simulink subsystem "Control_Motores"  (R2023b)
settings: Solver=VariableStepAuto  StartTime=0.0  StopTime=10.0  RelTol=1e-3
settings Model: Creator=Felix  LastModifiedBy=Felix

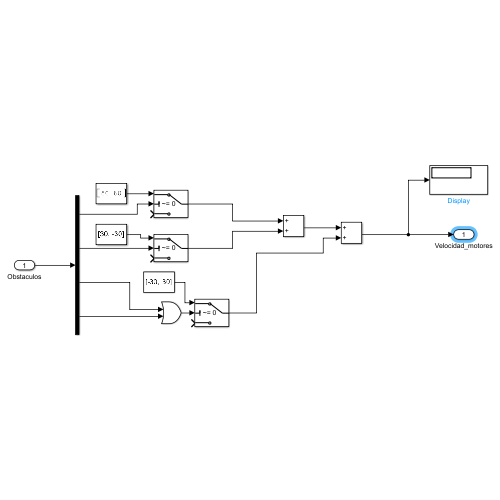
[thumbnail: Simulink's stored preview of the top-level diagram]
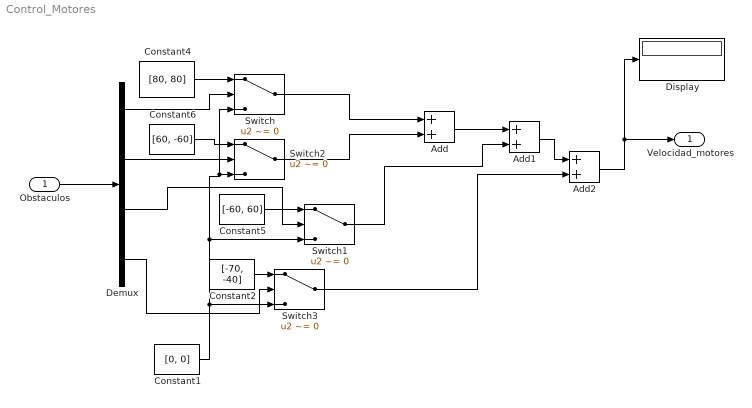
== system Control_Motores ==
  Obstaculos : Inport
  Add : Sum
  Add1 : Sum
  Add2 : Sum
  Constant1 : Constant  Value=[0, 0]  VectorParams1D=off
  Constant2 : Constant  Value=[-70, -40]  VectorParams1D=off
  Constant4 : Constant  Value=[80, 80]  VectorParams1D=off
  Constant5 : Constant  Value=[-60, 60]  VectorParams1D=off
  Constant6 : Constant  Value=[60, -60]  VectorParams1D=off
  Demux : Demux
  Display : Display
  Switch{,1..3} (4 alike) : Switch  Criteria=u2 ~= 0  SaturateOnIntegerOverflow=off  InputSameDT=off
  Velocidad_motores : Outport
  wires:
  Switch2/1 -> Add/2
  Switch/1 -> Add/1
  Add/1 -> Add1/1
  Constant6/1 -> Switch2/1
  Switch1/1 -> Add1/2
  Demux/4 -> Switch3/2
  Constant4/1 -> Switch/1
  Constant5/1 -> Switch1/1
  Demux/2 -> Switch2/2
  Demux/3 -> Switch1/2
  Demux/1 -> Switch/2
  Obstaculos/1 -> Demux/1
  Constant1/1 -> Switch1/3, Switch/3, Switch2/3, Switch3/3
  Constant2/1 -> Switch3/1
  Switch3/1 -> Add2/2
  Add1/1 -> Add2/1
  Add2/1 -> Velocidad_motores/1, Display/1
